simulink model "v1bate3"  (Simulink 8.8)
settings: Solver=ode3  StartTime=0.0  StopTime=inf  FixedStep=0.001  RelTol=1e-3  EnableMultiTasking=on
undefined symbols (not defined in the file): mdaadlink6208
libraries: simulink x19
(part 1 of 2)
settings Model: Creator=sayun  LastModifiedBy=lenovo  SimulationMode=external
settings SolverCC: EnableConcurrentExecution=on
settings OptimizationCC: BlockReduction=off  OptimizeBlockIOStorage=off  BufferReuse=off  GlobalBufferReuse=off  ExpressionFolding=off  ExpressionDepthLimit=2147483647  LocalBlockOutputs=off  LifeSpan=auto
settings DebuggingCC: SolverPrmCheckMsg=warning
settings HardwareCC: ProdIntDivRoundTo=Zero  ProdEndianess=LittleEndian  ProdLongLongMode=on  ProdHWDeviceType=Generic->32-bit x86 compatible
settings RTWCC: SystemTargetFile=slrt.tlc  TemplateMakefile=slrt_default_tmf  Description=Simulink Real-Time  RTWCompilerOptimization=on
settings SimulinkRealTimeCC: RL32LogBufSizeModifier=10000000

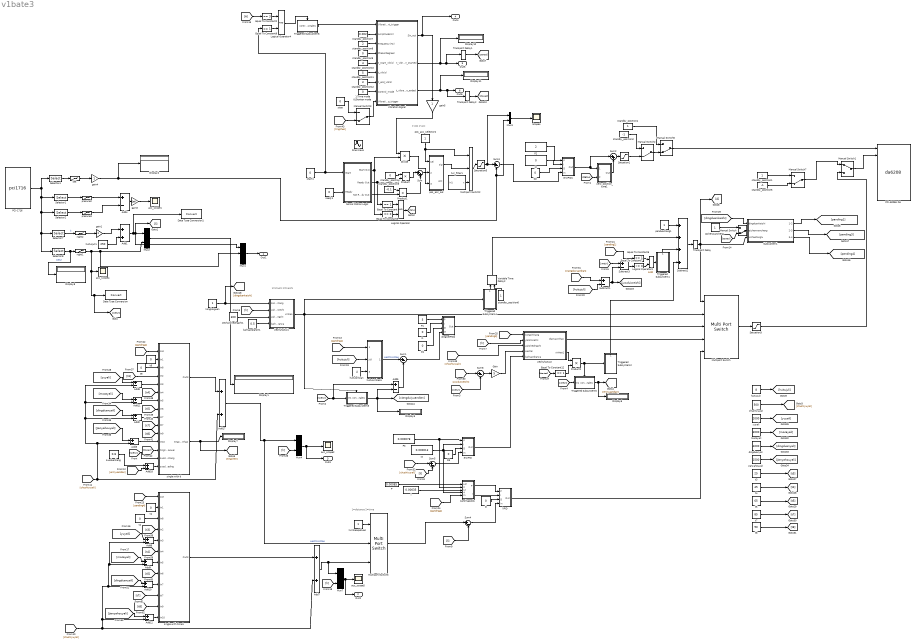
== system v1bate3 ==
  note: 1=chushi
      | 2=kaishi
  note: 1-pos
      | 2-acc
  note: 1=distance
      | 2=time
  1:Time mode 0:Shorten mode : Constant  Tag=kaognzhi  Description=kaognzhi  Value=0
  Add{1,7,17..18} (4 alike) : Sum
  Add{2..6,8..12} (10 alike) : Sum  Inputs=+-
  D{,1..3} (4 alike) : Constant  Value=0
  Data Type Conversion : DataTypeConversion
  Data Type Conversion1 : DataTypeConversion
  Display{1..2,5..8,10..11} (8 alike) : Display
  Divide : Product  Inputs=**
  Equal To Constant{,6,9,12} (4 alike) : simulink/Logic and Bit Operations/Compare To Constant  relop===  const=1  OutDataTypeStr=uint8  ZeroCross=off
  Equal To Constant2 : simulink/Logic and Bit Operations/Compare To Constant  relop===  const=3  OutDataTypeStr=uint8  ZeroCross=off
  Equal To Constant5 : simulink/Logic and Bit Operations/Compare To Constant  relop===  const=0  OutDataTypeStr=uint8  ZeroCross=off
  Equal To Constant7 : simulink/Logic and Bit Operations/Compare To Constant  relop=<=  const=0  OutDataTypeStr=uint8  ZeroCross=off
  Gain : Gain  Gain=5
  I : Constant  Value=0.00035
  I1 : Constant  Value=0
  I2 : Constant  Value=0
  I3 : Constant  Value=0.000013
  Logical Operator : Logic  AllPortsSameDT=off
  Logical Operator3 : Logic  AllPortsSameDT=off
  Logical Operator4 : Logic  AllPortsSameDT=off
  Manual Switch{,2..3,6..7} (5 alike) : ManualSwitch  CurrentSetting=0
  Manual Switch1 : ManualSwitch
  Multiport Switch : MultiPortSwitch  Inputs=4
  Multiport Switch2 : MultiPortSwitch  Inputs=2  SaturateOnIntegerOverflow=on
  Multiport Switch3 : MultiPortSwitch  Inputs=2
  Mux1 : Mux  Inputs=3
  Mux{2..4,7} (4 alike) : Mux  Inputs=2
  Nomal Motion Logic : Subsystem  AncestorBlock=control_logic_lib/Control Logic(Stateflow Chart)
  P : Constant  Value=0.00085
  P1 : Constant  Value=5
  P2 : Constant  Value=2
  P3 : Constant  Value=0.000078
  PCI-1716 : S-Function  FunctionName=pci1716  Parameters=[SampleTime SampleOffset], SLOT  SFunctionDeploymentMode=off  EnableBusSupport=off  mask(hitad3){Sample=0.001, SLOT=-1}
      mask prompts: Sample "Sample Time:"
      mask help:
      | PCi1716
      | A/D Card
      | Developed by ZhaoJinsong
      | 2012.06.02
      mask init:
      | SampleTime = 0.001; SampleOffset=0;
      mask Help: helpview([docroot '/toolbox/xpc/pt_io_block_reference.html#xpcioref'])
      mask Display:
      | disp('PCI1716  ');
      | 
      | port_label('output',1 , 'OUT');
  "PCI-6208A DA " : S-Function  InitFcn=mdaadlink6208( 1 );  FunctionName=da6208  Parameters=channel, range, sampletime, pcislot, reset, initval  SFunctionDeploymentMode=off  EnableBusSupport=off  mask(da6208){channel=[1:8], range=4 to 20 ma, reset=[0], initval=[0], sampletime=0.001, pcislot=-1}
      mask prompts: channel "Channel vector:"; reset "Reset vector:"; initval "Initial value vector:"; sampletime "Sample time:"; pcislot "PCI slot (-1: autosearch):"
      mask help:
      | PCI-6208A
      | Adlink
      | Analog Output
      mask init:
      | [maskdisplay, reset, initval]= mdaadlink6208(2, channel, reset, initval, pcislot);
      | set_param(gcb,'MaskDisplay',maskdisplay);
      mask Help: helpview(fullfile(docroot, 'mapfiles', 'xpc.map'), 'Adlink_6208A_DA')
      mask TypeOptions range: 0 to 20 ma | 5 to 25 ma | 4 to 20 ma
      mask Display: disp('PCI-6208A\nAdlink\nAnalog Output');port_label('input',1,'1');port_label('input',2,'2');port_label('input',3,'3');port_label('input',4,'4');port_label('input',5,'5');port_label('input',6,'6');port_label('input',7,'7');port_label('input',8,'8');
  Product : Product  SaturateOnIntegerOverflow=on  OutDataTypeStr=Inherit: Same as first input
  Product1 : Product  SaturateOnIntegerOverflow=on  OutDataTypeStr=Inherit: Same as first input
  Product2 : Product  RndMeth=Zero
  Satuation1 : Saturate  UpperLimit=10  LowerLimit=-10
  Satuation3 : Saturate  UpperLimit=10  LowerLimit=-10
  Saturation5 : Saturate  UpperLimit=10  LowerLimit=-10
  Scope4 : Scope
  Selector1 : Selector  IndexOptions=Index vector (dialog)  Indices=[3]  OutputSizes=1
  Selector2 : Selector  IndexOptions=Index vector (dialog)  Indices=[7]  OutputSizes=1
  Selector4 : Selector  IndexOptions=Index vector (dialog)  Indices=[1]  OutputSizes=1
  Selector7 : Selector  IndexOptions=Index vector (dialog)  Indices=[13]  OutputSizes=1
  Selector8 : Selector  IndexOptions=Index vector (dialog)  Indices=[15]  OutputSizes=1
  Sine Wave : Sin  Amplitude=0.001  Frequency=2*1*pi  SampleTime=0
  Subsystem1 : Subsystem
  Subtract1 : Sum  Inputs=+-
  Subtract2 : Sum  Inputs=++++
  Subtract3 : Sum  Inputs=+-
  Sum : Sum  Inputs=|++  SaturateOnIntegerOverflow=on
  Sum{1,4..5,8} (4 alike) : Sum  Inputs=|+-
  Sum2 : Sum  Inputs=|++  SaturateOnIntegerOverflow=on
  Sum3 : Sum  Inputs=|+-  SaturateOnIntegerOverflow=on
  Transport Delay : TransportDelay  DelayTime=0.0005
  Transport Delay1 : TransportDelay  DelayTime=0.0005
  Transport Delay2 : TransportDelay  DelayTime=0.0005
  Triggered Subsystem1 : Subsystem  TreatAsAtomicUnit=on
  Triggered Subsystem2 : Subsystem  TreatAsAtomicUnit=on
  Triggered Subsystem3 : Subsystem  TreatAsAtomicUnit=on
  Triggered Subsystem4 : Subsystem  TreatAsAtomicUnit=on
  Triggered Subsystem5 : Subsystem  TreatAsAtomicUnit=on
  Triggered Subsystem6 : Subsystem  TreatAsAtomicUnit=on
  Variable Time Delay2 : VariableTransportDelay  MaximumDelay=10
  Vibration Signal : Subsystem  TreatAsAtomicUnit=on
  acc_scope{1..2,4..5} (4 alike) : Scope
  canshuguodu : Subsystem
  chushiyuyali : Constant  Value=500
  dingduanyali : Constant  Value=4000
  dingweiPID2 : Subsystem
  erciPID : Subsystem
  erciPID1 : Subsystem
  gain1 : Gain  SaturateOnIntegerOverflow=on  OutDataTypeStr=Inherit: Same as input  ParamDataTypeStr=Inherit: Same as input
  gain3 : Gain  Gain=1e6  SaturateOnIntegerOverflow=on  OutDataTypeStr=Inherit: Same as input  ParamDataTypeStr=Inherit: Same as input
  gain4 : Gain  SaturateOnIntegerOverflow=on  OutDataTypeStr=Inherit: Same as input  ParamDataTypeStr=Inherit: Same as input
  gain5 : Gain  SaturateOnIntegerOverflow=on  OutDataTypeStr=Inherit: Same as input  ParamDataTypeStr=Inherit: Same as input
  huituijuli : Constant  Value=8
  huituijuli1 : Constant  Value=250
  huituishijian : Constant  Value=4
  huituixinhao1 : Subsystem
  jianyahouyali : Constant  Value=1500
  jiechuhuitui1 : Subsystem
  jiechuhuitui2 : Subsystem
  jiechulishedingzhi1 : Constant  Value=300
  kaihuanqianjin1 : Constant  Value=0.5
  left : Lookup  InputValues=[2.090 9.905]  Table=[-10 10]  SaturateOnIntegerOverflow=on
  liPID : Subsystem
  lixinhaoqiehuan : Constant
      settings: OpenFcn=|
      | if get_param(gcb,'value')=='1',
      | set_param(gcb,'value','2');
      | else
      | set_param(gcb,'value','1');end
  mocayali : Constant  Value=3000
  panduanliang1 : Constant
  pos_acc_sel : Subsystem
  pos_acc_selector2 : Constant
      settings: OpenFcn=|
      | if get_param(gcb,'value')=='1',
      | set_param(gcb,'value','2');
      | else
      | set_param(gcb,'value','1');end
  presure2 : Lookup  InputValues=[2 10]  Table=[0 25]  SaturateOnIntegerOverflow=on
  presure3 : Lookup  InputValues=[2 10]  Table=[0 25]  SaturateOnIntegerOverflow=on
  qizhenwancheng : Constant
      settings: OpenFcn=|
      | if get_param(gcb,'value')=='1',
      | set_param(gcb,'value','0');
      | else
      | set_param(gcb,'value','1');end
  ready1 : Constant  Value=0
      settings: OpenFcn=|
      | if get_param(gcb,'value')=='1',
      | set_param(gcb,'value','0');
      | else
      | set_param(gcb,'value','1');end
  right1 : Lookup  InputValues=[1.264 5.214]  Table=[0 20]  SaturateOnIntegerOverflow=on
  right2 : Lookup  InputValues=[2 10]  Table=[-29400 29400]  SaturateOnIntegerOverflow=on
  single with d : Subsystem
  single with time1 : Subsystem
  standby_position : Constant  Value=0
  standby_position1 : Constant
  standby_position10 : Constant  Value=4
  standby_position11 : Constant  Value=5
  standby_position12 : Constant  Value=3
  standby_position2 : Constant  Value=-1
  standby_position3 : Constant  Value=-0.1
  standby_position4 : Constant
  standby_position5 : Constant  Value=-1
  standby_position6 : Constant
  standby_position7 : Constant  Value=0.002
  standby_position8 : Constant  Value=2
  standby_position9 : Constant  Value=0
  start1 : Constant  Value=0
      settings: OpenFcn=|
      | if get_param(gcb,'value')=='1',
      | set_param(gcb,'value','0');
      | else
      | set_param(gcb,'value','1');end
  stop : Constant  Value=0
      settings: OpenFcn=|
      | if get_param(gcb,'value')=='1',
      | set_param(gcb,'value','0');
      | else
      | set_param(gcb,'value','1');end
  suoduanliang : Constant  Value=0.8
  t{1..2,6,9} (4 alike) : Constant  Value=0
  t3 : Constant  Value=25
  t4 : Constant  Value=45
  t5 : Constant  Value=65
  t7 : Constant  Value=85
  t8 : Constant  Value=90
  tvc_filter1 : Subsystem
      mask Display: disp('Reference\nModule')
  yuyali : Constant  Value=2000
  zero_position_tune1 : Subsystem
  zongkaiguan : Constant
      settings: OpenFcn=|
      | if get_param(gcb,'value')=='1',
      | set_param(gcb,'value','2');
      | else
      | set_param(gcb,'value','1');end
  Out1 : Outport
  Out2 : Outport  Port=2
  Out3 : Outport  Port=3
  Out4 : Outport  Port=4
  Out5 : Outport  Port=5
  Out6 : Outport  Port=6
  tag scope: status=global
  wires:
  kaihuanqianjin1/1 -> jiechuhuitui1/4(kaihuandianya)
  jiechulishedingzhi1/1 -> jiechuhuitui1/3(yalishedingzhi)
  jiechuhuitui1/1(xinhao) -> Triggered Subsystem4/Trigger, Triggered Subsystem3/Trigger, Multiport Switch/2
  huituishijian/1 -> huituixinhao1/3(shijian)
  [huitujuli] -> huituixinhao1/2(juli)
  panduanliang1/1 -> Subtract2/1
  Variable Time Delay2/1 -> Subtract2/2
  Equal To Constant7/1 -> Logical Operator3/2
  Equal To Constant6/1 -> Logical Operator3/1
  Subtract3/1 -> Equal To Constant7/1
  huituixinhao1/1(Out2) -> Sum1/1  "weizhixinhao"
  Sum1/1 -> dingweiPID2/4(In)
  zongkaiguan/1 -> [dingduankaishi], jiechuhuitui1/1(kongzhiliang)
  left/1 -> gain4/1
  PCI-1716/1 -> Selector4/1, Selector1/1, Selector2/1, Selector7/1, Selector8/1
  Selector4/1 -> left/1
  Selector1/1 -> presure2/1
  Selector2/1 -> presure3/1
  presure2/1 -> Add4/1
  presure3/1 -> Add4/2
  Add4/1 -> gain3/1
  gain3/1 -> acc_scope1/1
  Mux2/1 -> Display1/1
  Selector7/1 -> right2/1  "li"
  Selector8/1 -> right1/1, Display8/1  "weiyi"
  right2/1 -> gain1/1
  right1/1 -> Mux2/2, Mux1/2, acc_scope4/1, Data Type Conversion/1, [weiyi]
  gain1/1 -> Add1/1
  ready1/1 -> Nomal Motion Logic/2(Ready)
  start1/1 -> Nomal Motion Logic/1(Start), Equal To Constant9/1
  Nomal Motion Logic/2(Ready Out) -> Equal To Constant/1, Product/2
  standby_position/1 -> Product/1
  Product/1 -> Sum/1
  Sum/1 -> pos_acc_sel/3(ini_pos)
  Nomal Motion Logic/1(Start Out) -> Divide/2, Equal To Constant5/1
  Equal To Constant/1 -> Logical Operator/1
  Logical Operator/1 -> [status]
  pos_acc_selector2/1 -> pos_acc_sel/1(sel), Multiport Switch2/1
  Nomal Motion Logic/3(Not Ready Out) -> Product1/2
  standby_position3/1 -> Product1/1
  Product1/1 -> Sum/2
  Multiport Switch2/1 -> Saturation5/1
  [status] -> zero_position_tune1/2(status)
  pos_acc_sel/1(sig) -> Multiport Switch2/2
  zero_position_tune1/1(Out) -> Sum2/2
  Sum2/1 -> Satuation1/1
  Sum3/1 -> erciPID1/4(In)
  tvc_filter1/1(x) -> Multiport Switch2/3
  Satuation1/1 -> Manual Switch2/2
  standby_position2/1 -> Manual Switch2/1
  Saturation5/1 -> Sum3/1, Mux3/1
  Manual Switch2/1 -> Manual Switch6/2
  standby_position4/1 -> Manual Switch6/1
  Divide/1 -> pos_acc_sel/2(sig_in)
  erciPID1/1(Out) -> Sum2/1, zero_position_tune1/1(error_in)
  Mux3/1 -> Scope4/1
  Equal To Constant5/1 -> Logical Operator/2
  Manual Switch6/1 -> "PCI-6208A DA "/1
  gain4/1 -> Sum3/2, Mux3/2, Display2/1
  standby_position1/1 -> Manual Switch7/1
  standby_position5/1 -> Manual Switch7/2
  dingweiPID2/1(Out) -> Multiport Switch/3
  huituijuli1/1 -> Add1/2
  Add1/1 -> Data Type Conversion1/1, Mux2/1, [li], Mux1/1
  Mux1/1 -> Out1/1
  Transport Delay/1 -> [A], Subsystem1/3(xinhaotonglu), Multiport Switch/1
  Add5/1 -> Sum1/2
  chushiyuyali/1 -> [chushiyuyali]
  lixinhaoqiehuan/1 -> Multiport Switch3/1
  Logical Operator3/1 -> Triggered Subsystem1/Trigger
  Triggered Subsystem1/1(control-single1) -> Subtract2/3
  Product2/1 -> Triggered Subsystem2/Trigger, Triggered Subsystem5/Trigger
  single with time1/1(Out3) -> Add7/1
  Add7/1 -> Mux7/1, Multiport Switch3/3
  Triggered Subsystem2/1(control-single1) -> Subtract2/4
  canshuguodu/1(P) -> liPID/1(P)
  [yuyali] -> Add6/1
  Add6/1 -> single with time1/5(In3)
  Add9/1 -> single with time1/7(In5)
  Add10/1 -> single with time1/9(In7)
  P3/1 -> erciPID/1(P), canshuguodu/2(erciP)
  t1/1 -> single with time1/2(In1)
  t2/1 -> single with time1/3(In8)
  Add12/1 -> single with time1/12(In10)
  jiechuhuitui2/2(xinhao1) -> Product2/1
  I3/1 -> erciPID/2(I), canshuguodu/4(erciI)
  P/1 -> canshuguodu/1(LiP)
  I/1 -> canshuguodu/3(LiI)
  canshuguodu/2(I) -> liPID/2(I)
  Subtract1/1 -> Subtract3/2, [juwduiweizhi]
  Triggered Subsystem4/1(control-single1) -> Variable Time Delay2/1
  standby_position6/1 -> Variable Time Delay2/2
  t6/1 -> single with d/2(In1)
  single with d/1(Out3) -> Add17/1
  t9/1 -> single with d/3(In8)
  [stoped] -> single with d/13(tingzhendaowei)
  Add18/1 -> single with d/15(suoduanliangsheding)
  suoduanliang/1 -> Add18/1
  single with d/2(tingzhenxinhao) -> Display7/1, [tingzhen]
  Gain/1 -> jiechuhuitui2/4(wentai)
  Sum8/1 -> Gain/1
  standby_position7/1 -> Vibration Signal/2(Amplitude(m))
  standby_position8/1 -> Vibration Signal/3(Frequency(Hz))
  standby_position9/1 -> Vibration Signal/4(Phase(Degree))
  standby_position10/1 -> Vibration Signal/5(t_start_vib(s))
  Triggered Subsystem6/1(control-single1) -> Vibration Signal/1(Vibration_start_trigger)
  standby_position11/1 -> Vibration Signal/6(t_vib(s))
  standby_position12/1 -> Vibration Signal/7(t_end_vib(s))
  Vibration Signal/1(Sin_out) -> Out4/1, gain5/1
  Vibration Signal/2(t_vibration_started) -> Display10/1, Out5/1, Transport Delay1/1
  Vibration Signal/3(t_vibration_ended) -> Display11/1, Out6/1, Transport Delay2/1
  1:Time mode 0:Shorten mode/1 -> Vibration Signal/8(Control_mode)
  [weiyi] -> single with d/14(suoduanliang)
  [weiyi] -> Triggered Subsystem3/1(In1), Add5/1
  [weiyi] -> Sum8/2
  [weiyi] -> Triggered Subsystem5/1(In1)
  [weiyi] -> Subtract3/1
  [li] -> jiechuhuitui1/2(yalishicezhi)
  [li] -> jiechuhuitui2/2(yalishicezhi)
  [li] -> Sum5/2
  erciPID/1(Out) -> jiechuhuitui2/5(kaihuandianya)
  D3/1 -> erciPID/3(D)
  D/1 -> liPID/3(D)
  [chushiyuyali] -> Add7/2, Add12/2, Add10/2, Add9/2, Add6/2
  [chushiyuyali] -> Add17/2, Add3/2, Add2/2, Add11/2, Add8/2
  [erciyuandian] -> Add18/2
  gain5/1 -> Divide/1
  qizhenwancheng/1 -> Manual Switch/1
  [started] -> Manual Switch/2
  [A] -> Equal To Constant2/1
  Equal To Constant2/1 -> Logical Operator4/1
  Equal To Constant9/1 -> Logical Operator4/2
  Logical Operator4/1 -> Triggered Subsystem6/Trigger
  P2/1 -> erciPID1/1(P)
  I2/1 -> erciPID1/2(I)
  D2/1 -> erciPID1/3(D)
  huituijuli/1 -> [huitujuli]
  [huitujuli] -> Subtract1/2
  [panding4] -> single with d/1(con)
  [panding4] -> single with time1/1(con)
  [panding4] -> canshuguodu/5(In)
  [panding3] -> jiechuhuitui2/1(kongzhiliang)
  [started] -> Equal To Constant12/1
  Equal To Constant12/1 -> Product2/2
  [dingduankaishi] -> Subsystem1/1(dingduankaishi)
  Manual Switch/1 -> Subsystem1/2(qizhenwancheng)
  Subtract2/1 -> Transport Delay/1
  [juwduiweizhi] -> Sum8/1
  P1/1 -> dingweiPID2/1(P)
  I1/1 -> dingweiPID2/2(I)
  D1/1 -> dingweiPID2/3(D)
  [xiangduiyuandian] -> Subtract1/1
  Triggered Subsystem5/1(control-single1) -> [erciyuandian], Display6/1
  Triggered Subsystem3/1(control-single1) -> Add5/2, [xiangduiyuandian], Display5/1
  [chushiyuyali] -> Sum5/1
  [chushiyuyali] -> jiechuhuitui2/3(yalishedingzhi)
  Sum5/1 -> erciPID/4(In)
  ? -> ?
  [t3] -> single with time1/4(In2)
  [mocayali] -> Add9/1
  [dingduanyali] -> Add10/1
  [jianyahouyali] -> Add12/1
  [li] -> Sum4/2
  Sum4/1 -> liPID/4(In)
  Multiport Switch3/1 -> Sum4/1
  Mux7/1 -> acc_scope5/1, Out2/1
  [li] -> Mux7/2
  Mux4/1 -> acc_scope2/1, Out3/1
  [li] -> Mux4/2
  [t4] -> single with time1/6(In4)
  [t5] -> single with time1/8(In6)
  [t7] -> single with time1/10(tt7)
  [t8] -> single with time1/11(In9)
  [yuyali] -> Add8/1
  [mocayali] -> Add11/1
  [dingduanyali] -> Add2/1
  [jianyahouyali] -> Add3/1
  Add3/1 -> single with d/12(In10)
  [t3] -> single with d/4(In2)
  Add8/1 -> single with d/5(In3)
  [t4] -> single with d/6(In4)
  Add11/1 -> single with d/7(In5)
  [t5] -> single with d/8(In6)
  Add2/1 -> single with d/9(In7)
  [t7] -> single with d/10(tt7)
  [t8] -> single with d/11(In9)
  Add17/1 -> Mux4/1, Multiport Switch3/2  "weizhixinhao"
  yuyali/1 -> [yuyali]
  mocayali/1 -> [mocayali]
  dingduanyali/1 -> [dingduanyali]
  jianyahouyali/1 -> [jianyahouyali]
  t3/1 -> [t3]
  t4/1 -> [t4]
  t5/1 -> [t5]
  t7/1 -> [t7]
  t8/1 -> [t8]
  Manual Switch7/1 -> Manual Switch1/1
  [panding1] -> Equal To Constant6/1
  Subsystem1/1(1-2) -> [panding1]
  Subsystem1/2(2-3) -> [panding3]
  Subsystem1/3(3-4) -> [panding4]
  Multiport Switch/1 -> Satuation3/1
  jiechuhuitui2/1(dianyaxinhao) -> Multiport Switch/4
  [panding1] -> huituixinhao1/1(con1)
  liPID/1(Out) -> Multiport Switch/5
  Manual Switch1/1 -> "PCI-6208A DA "/2
  Satuation3/1 -> Manual Switch1/2
  Manual Switch3/1 -> Vibration Signal/9(Vibration_stop_trigger)
  stop/1 -> Manual Switch3/1
  [tingzhen] -> Manual Switch3/2
  Transport Delay2/1 -> [stoped]
  Transport Delay1/1 -> [started]

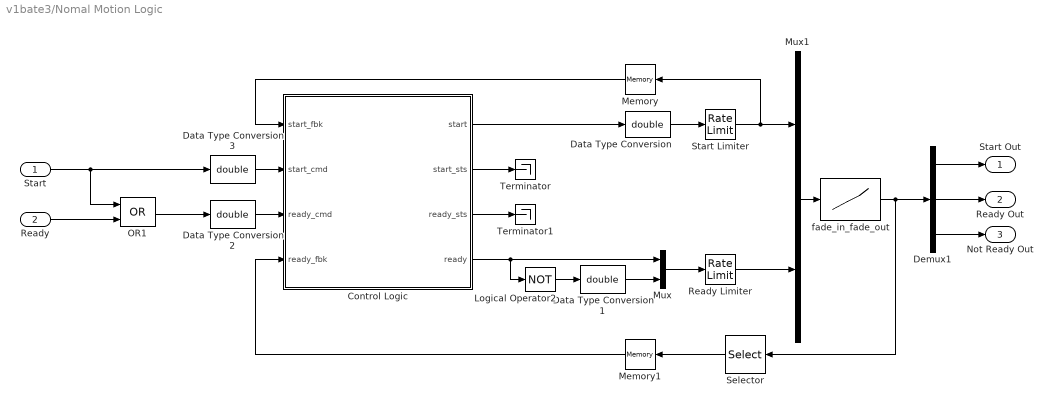
== system v1bate3/Nomal Motion Logic ==
  Start : Inport
  Ready : Inport  Port=2
  Control Logic : Stateflow chart  TreatAsAtomicUnit=on
  Data Type Conversion{,1..3} (4 alike) : DataTypeConversion  OutDataTypeStr=double  SaturateOnIntegerOverflow=on  RndMeth=Zero
  Demux1 : Demux  Outputs=3
  Logical Operator2 : Logic  Operator=NOT  Inputs=3  AllPortsSameDT=off
  Memory : Memory
  Memory1 : Memory
  Mux : Mux  Inputs=2
  Mux1 : Mux  Inputs=2
  OR1 : Logic  Operator=OR  AllPortsSameDT=off
  Ready Limiter : RateLimiter  RisingSlewLimit=1/5  FallingSlewLimit=-1/5
  Selector : Selector  InputPortWidth=3  IndexOptions=Index vector (dialog)  Indices=[2]  OutputSizes=1
  Start Limiter : RateLimiter  RisingSlewLimit=1/3  FallingSlewLimit=-1/3
  Terminator : Terminator
  Terminator1 : Terminator
  fade_in_fade_out : Lookup  InputValues=[0:0.001:1]  Table=(sin(([0:0.001:1]*2-1)*pi/2)+1)/2  SaturateOnIntegerOverflow=on
  Start Out : Outport
  Ready Out : Outport  Port=2
  Not Ready Out : Outport  Port=3
  wires:
  Ready/1 -> OR1/2
  Start/1 -> OR1/1, Data Type Conversion3/1
  Control Logic/3(ready_sts) -> Terminator1/1
  Control Logic/2(start_sts) -> Terminator/1
  OR1/1 -> Data Type Conversion2/1
  Data Type Conversion3/1 -> Control Logic/2(start_cmd)
  Demux1/3 -> Not Ready Out/1
  Demux1/1 -> Start Out/1
  Demux1/2 -> Ready Out/1
  Data Type Conversion/1 -> Start Limiter/1
  Start Limiter/1 -> Mux1/1, Memory/1
  Control Logic/1(start) -> Data Type Conversion/1
  Control Logic/4(ready) -> Logical Operator2/1, Mux/1
  Logical Operator2/1 -> Data Type Conversion1/1
  Mux/1 -> Ready Limiter/1
  Ready Limiter/1 -> Mux1/2
  Mux1/1 -> fade_in_fade_out/1
  fade_in_fade_out/1 -> Selector/1, Demux1/1
  Memory/1 -> Control Logic/1(start_fbk)
  Memory1/1 -> Control Logic/4(ready_fbk)
  Data Type Conversion1/1 -> Mux/2
  Data Type Conversion2/1 -> Control Logic/3(ready_cmd)
  Selector/1 -> Memory1/1

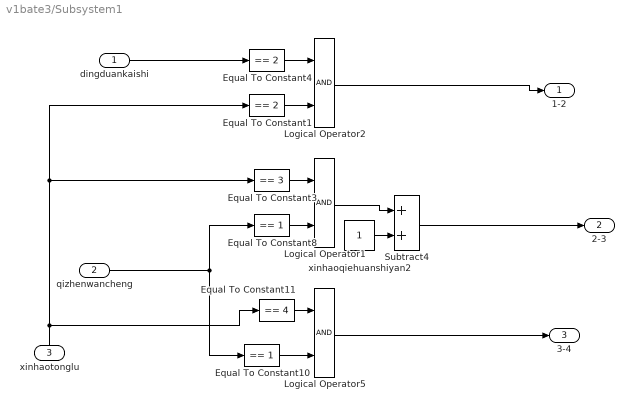
== system v1bate3/Subsystem1 ==
  dingduankaishi : Inport
  qizhenwancheng : Inport  Port=2
  xinhaotonglu : Inport  Port=3
  Equal To Constant1 : simulink/Logic and Bit Operations/Compare To Constant  relop===  const=2  OutDataTypeStr=uint8  ZeroCross=off
  Equal To Constant10 : simulink/Logic and Bit Operations/Compare To Constant  relop===  const=1  OutDataTypeStr=uint8  ZeroCross=off
  Equal To Constant11 : simulink/Logic and Bit Operations/Compare To Constant  relop===  const=4  OutDataTypeStr=uint8  ZeroCross=off
  Equal To Constant3 : simulink/Logic and Bit Operations/Compare To Constant  relop===  const=3  OutDataTypeStr=uint8  ZeroCross=off
  Equal To Constant4 : simulink/Logic and Bit Operations/Compare To Constant  relop===  const=2  OutDataTypeStr=uint8  ZeroCross=off
  Equal To Constant8 : simulink/Logic and Bit Operations/Compare To Constant  relop===  const=1  OutDataTypeStr=uint8  ZeroCross=off
  Logical Operator1 : Logic  AllPortsSameDT=off
  Logical Operator2 : Logic  AllPortsSameDT=off
  Logical Operator5 : Logic  AllPortsSameDT=off
  Subtract4 : Sum
  xinhaoqiehuanshiyan2 : Constant
  1-2 : Outport
  2-3 : Outport  Port=2
  3-4 : Outport  Port=3
  wires:
  Equal To Constant4/1 -> Logical Operator2/1
  Equal To Constant1/1 -> Logical Operator2/2
  Equal To Constant3/1 -> Logical Operator1/1
  Equal To Constant8/1 -> Logical Operator1/2
  xinhaoqiehuanshiyan2/1 -> Subtract4/2
  Logical Operator1/1 -> Subtract4/1
  Equal To Constant11/1 -> Logical Operator5/1
  Equal To Constant10/1 -> Logical Operator5/2
  qizhenwancheng/1 -> Equal To Constant10/1, Equal To Constant8/1
  xinhaotonglu/1 -> Equal To Constant11/1, Equal To Constant3/1, Equal To Constant1/1
  dingduankaishi/1 -> Equal To Constant4/1
  Logical Operator2/1 -> 1-2/1
  Subtract4/1 -> 2-3/1
  Logical Operator5/1 -> 3-4/1

== system v1bate3/Triggered Subsystem1 ==
  Trigger : TriggerPort  VariantControl=Variant
  Constant : Constant
  control-single1 : Outport
  wires:
  Constant/1 -> control-single1/1

== system v1bate3/Triggered Subsystem2 ==
  Trigger : TriggerPort  VariantControl=Variant
  Constant : Constant
  control-single1 : Outport
  wires:
  Constant/1 -> control-single1/1

== system v1bate3/Triggered Subsystem3 ==
  In1 : Inport
  Trigger : TriggerPort  TriggerType=falling  VariantControl=Variant
  control-single1 : Outport
  wires:
  In1/1 -> control-single1/1

== system v1bate3/Triggered Subsystem4 ==
  Trigger : TriggerPort  TriggerType=falling  VariantControl=Variant
  Constant : Constant
  control-single1 : Outport
  wires:
  Constant/1 -> control-single1/1

== system v1bate3/Triggered Subsystem5 ==
  In1 : Inport
  Trigger : TriggerPort  VariantControl=Variant
  control-single1 : Outport
  wires:
  In1/1 -> control-single1/1

== system v1bate3/Triggered Subsystem6 ==
  Trigger : TriggerPort  VariantControl=Variant
  Constant : Constant
  control-single1 : Outport
  wires:
  Constant/1 -> control-single1/1

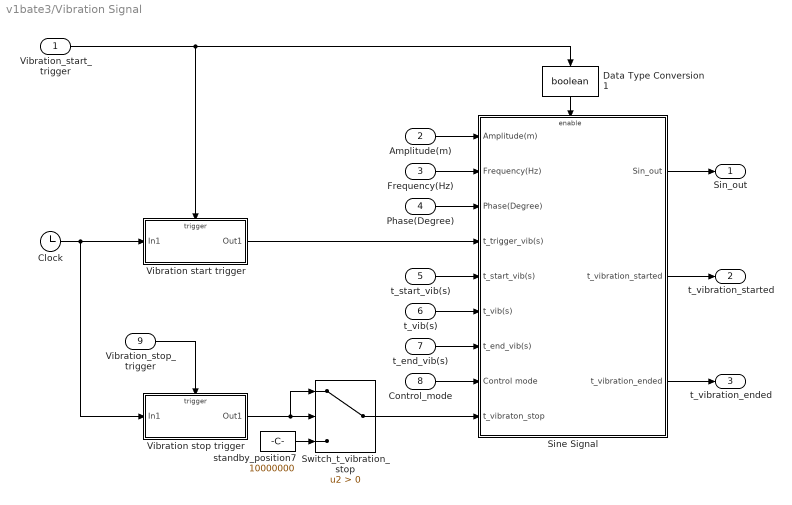
== system v1bate3/Vibration Signal ==
  Vibration_start_trigger : Inport
  Amplitude(m) : Inport  Port=2
  Frequency(Hz) : Inport  Port=3
  Phase(Degree) : Inport  Port=4
  t_start_vib(s) : Inport  Port=5
  t_vib(s) : Inport  Port=6
  t_end_vib(s) : Inport  Port=7
  Control_mode : Inport  Port=8
  Vibration_stop_trigger : Inport  Port=9
  Clock : Clock
  Data Type Conversion1 : DataTypeConversion  OutDataTypeStr=boolean  SaturateOnIntegerOverflow=on  RndMeth=Zero
  Sine Signal : Subsystem
  Switch_t_vibration_stop : Switch  Criteria=u2 > Threshold
  Vibration start trigger : Subsystem  TreatAsAtomicUnit=on
  Vibration stop trigger : Subsystem  TreatAsAtomicUnit=on
  standby_position7 : Constant  Value=10000000
  Sin_out : Outport
  t_vibration_started : Outport  Port=2
  t_vibration_ended : Outport  Port=3
  wires:
  Data Type Conversion1/1 -> Sine Signal/Enable
  Phase(Degree)/1 -> Sine Signal/3(Phase(Degree))
  Vibration_start_trigger/1 -> Data Type Conversion1/1, Vibration start trigger/Trigger
  Frequency(Hz)/1 -> Sine Signal/2(Frequency(Hz))
  Vibration start trigger/1(Out1) -> Sine Signal/4(t_trigger_vib(s))
  Clock/1 -> Vibration start trigger/1(In1), Vibration stop trigger/1(In1)
  Amplitude(m)/1 -> Sine Signal/1(Amplitude(m))
  t_start_vib(s)/1 -> Sine Signal/5(t_start_vib(s))
  t_vib(s)/1 -> Sine Signal/6(t_vib(s))
  t_end_vib(s)/1 -> Sine Signal/7(t_end_vib(s))
  Sine Signal/1(Sin_out) -> Sin_out/1
  Sine Signal/2(t_vibration_started) -> t_vibration_started/1
  Sine Signal/3(t_vibration_ended) -> t_vibration_ended/1
  Control_mode/1 -> Sine Signal/8(Control mode)
  Vibration_stop_trigger/1 -> Vibration stop trigger/Trigger
  standby_position7/1 -> Switch_t_vibration_stop/3
  Vibration stop trigger/1(Out1) -> Switch_t_vibration_stop/2, Switch_t_vibration_stop/1
  Switch_t_vibration_stop/1 -> Sine Signal/9(t_vibraton_stop)

== system v1bate3/canshuguodu ==
  LiP : Inport
  erciP : Inport  Port=2
  LiI : Inport  Port=3
  erciI : Inport  Port=4
  In : Inport  Port=5
  Nomal Motion Logic1 : Subsystem  AncestorBlock=control_logic_lib/Control Logic(Stateflow Chart)
  Nomal Motion Logic2 : Subsystem  AncestorBlock=control_logic_lib/Control Logic(Stateflow Chart)
  Product{12..15} (4 alike) : Product  SaturateOnIntegerOverflow=on  OutDataTypeStr=Inherit: Same as first input
  Sum6 : Sum  Inputs=|++  SaturateOnIntegerOverflow=on
  Sum7 : Sum  Inputs=|++  SaturateOnIntegerOverflow=on
  start4 : Constant  Value=0
      settings: OpenFcn=|
      | if get_param(gcb,'value')=='1',
      | set_param(gcb,'value','0');
      | else
      | set_param(gcb,'value','1');end
  start5 : Constant  Value=0
      settings: OpenFcn=|
      | if get_param(gcb,'value')=='1',
      | set_param(gcb,'value','0');
      | else
      | set_param(gcb,'value','1');end
  P : Outport
  I : Outport  Port=2
  wires:
  start4/1 -> Nomal Motion Logic1/1(Start)
  Nomal Motion Logic1/2(Ready Out) -> Product12/2
  Product12/1 -> Sum6/1
  Nomal Motion Logic1/3(Not Ready Out) -> Product13/2
  Product13/1 -> Sum6/2
  start5/1 -> Nomal Motion Logic2/1(Start)
  Nomal Motion Logic2/2(Ready Out) -> Product14/2
  Product14/1 -> Sum7/1
  Nomal Motion Logic2/3(Not Ready Out) -> Product15/2
  Product15/1 -> Sum7/2
  erciP/1 -> Product13/1
  In/1 -> Nomal Motion Logic2/2(Ready), Nomal Motion Logic1/2(Ready)
  erciI/1 -> Product15/1
  Nomal Motion Logic1/1(Start Out) -> ?
  LiP/1 -> Product12/1
  Sum6/1 -> P/1
  Nomal Motion Logic2/1(Start Out) -> ?
  LiI/1 -> Product14/1
  Sum7/1 -> I/1

== system v1bate3/dingweiPID2 ==
  P : Inport
  I : Inport  Port=2
  D : Inport  Port=3
  In : Inport  Port=4
  Add19 : Sum  Inputs=+++
  Derivative4 : Derivative
  Integrator5 : Integrator
  Product16 : Product  RndMeth=Zero
  Product17 : Product  RndMeth=Zero
  Product18 : Product  RndMeth=Zero
  Out : Outport
  wires:
  D/1 -> Product17/1
  Add19/1 -> Out/1
  I/1 -> Product16/1
  In/1 -> Product17/2, Product16/2, Product18/2
  P/1 -> Product18/1
  Product17/1 -> Derivative4/1
  Product16/1 -> Integrator5/1
  Product18/1 -> Add19/1
  Integrator5/1 -> Add19/2
  Derivative4/1 -> Add19/3

== system v1bate3/erciPID ==
  P : Inport
  I : Inport  Port=2
  D : Inport  Port=3
  In : Inport  Port=4
  Add19 : Sum  Inputs=+++
  Derivative4 : Derivative
  Integrator5 : Integrator
  Product16 : Product  RndMeth=Zero
  Product17 : Product  RndMeth=Zero
  Product18 : Product  RndMeth=Zero
  Out : Outport
  wires:
  Derivative4/1 -> Add19/3
  Integrator5/1 -> Add19/2
  Product18/1 -> Add19/1
  Product16/1 -> Integrator5/1
  Product17/1 -> Derivative4/1
  P/1 -> Product18/1
  In/1 -> Product18/2, Product16/2, Product17/2
  I/1 -> Product16/1
  Add19/1 -> Out/1
  D/1 -> Product17/1

== system v1bate3/erciPID1 ==
  P : Inport
  I : Inport  Port=2
  D : Inport  Port=3
  In : Inport  Port=4
  Add19 : Sum  Inputs=+++
  Derivative4 : Derivative
  Integrator5 : Integrator
  Product16 : Product  RndMeth=Zero
  Product17 : Product  RndMeth=Zero
  Product18 : Product  RndMeth=Zero
  Out : Outport
  wires:
  D/1 -> Product17/1
  Add19/1 -> Out/1
  I/1 -> Product16/1
  In/1 -> Product17/2, Product16/2, Product18/2
  P/1 -> Product18/1
  Product17/1 -> Derivative4/1
  Product16/1 -> Integrator5/1
  Product18/1 -> Add19/1
  Integrator5/1 -> Add19/2
  Derivative4/1 -> Add19/3

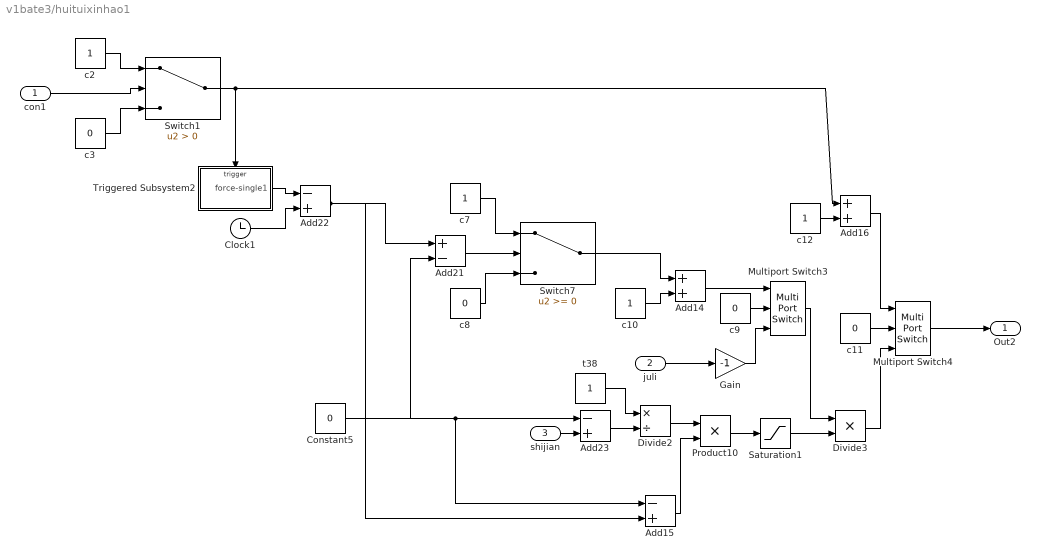
== system v1bate3/huituixinhao1 ==
  con1 : Inport
  juli : Inport  Port=2
  shijian : Inport  Port=3
  Add14 : Sum
  Add15 : Sum  Inputs=-+
  Add16 : Sum
  Add21 : Sum  Inputs=+-
  Add22 : Sum  Inputs=-+
  Add23 : Sum  Inputs=-+
  Clock1 : Clock
  Constant5 : Constant  Value=0
  Divide2 : Product  Inputs=*/
  Divide3 : Product  Inputs=**
  Gain : Gain  Gain=-1
  Multiport Switch3 : MultiPortSwitch  Inputs=2
  Multiport Switch4 : MultiPortSwitch  Inputs=2
  Product10 : Product  RndMeth=Zero
  Saturation1 : Saturate  UpperLimit=1  LowerLimit=-1
  Switch1 : Switch  Criteria=u2 > Threshold
  Switch7 : Switch
  Triggered Subsystem2 : Subsystem  TreatAsAtomicUnit=on
  c{2,7,10,12} (4 alike) : Constant
  c{3,8..9,11} (4 alike) : Constant  Value=0
  t38 : Constant
  Out2 : Outport
  wires:
  c12/1 -> Add16/2
  Multiport Switch4/1 -> Out2/1
  Add16/1 -> Multiport Switch4/1
  c11/1 -> Multiport Switch4/2
  shijian/1 -> Add23/2
  juli/1 -> Gain/1
  con1/1 -> Switch1/2
  Gain/1 -> Multiport Switch3/3
  Switch1/1 -> Add16/1, Triggered Subsystem2/Trigger
  c3/1 -> Switch1/3
  c2/1 -> Switch1/1
  Add22/1 -> Add15/2, Add21/1
  c10/1 -> Add14/2
  Switch7/1 -> Add14/1
  Add14/1 -> Multiport Switch3/1
  c9/1 -> Multiport Switch3/2
  Add21/1 -> Switch7/2
  c8/1 -> Switch7/3
  c7/1 -> Switch7/1
  Multiport Switch3/1 -> Divide3/1
  Constant5/1 -> Add21/2, Add15/1, Add23/1
  Add15/1 -> Product10/2
  Divide2/1 -> Product10/1
  Add23/1 -> Divide2/2
  Saturation1/1 -> Divide3/2
  Product10/1 -> Saturation1/1
  t38/1 -> Divide2/1
  Clock1/1 -> Add22/2
  Triggered Subsystem2/1(force-single1) -> Add22/1
  Divide3/1 -> Multiport Switch4/3

== system v1bate3/jiechuhuitui1 ==
  kongzhiliang : Inport
  yalishicezhi : Inport  Port=2
  yalishedingzhi : Inport  Port=3
  kaihuandianya : Inport  Port=4
  Add : Sum  Inputs=+-
  Add1 : Sum  Inputs=+-
  Multiport Switch : MultiPortSwitch
  Switch1 : Switch
  c2 : Constant  Value=-1
  c3 : Constant  Value=0
  chushi : Constant  Value=-1
  tingzhi : Constant  Value=0
  xinhao : Outport
  wires:
  chushi/1 -> Multiport Switch/2
  c2/1 -> Switch1/1
  c3/1 -> Switch1/3
  Add/1 -> Switch1/2
  tingzhi/1 -> Multiport Switch/4
  Switch1/1 -> Add1/2
  Add1/1 -> Multiport Switch/1
  kongzhiliang/1 -> Add1/1
  yalishicezhi/1 -> Add/1
  yalishedingzhi/1 -> Add/2
  kaihuandianya/1 -> Multiport Switch/3
  Multiport Switch/1 -> xinhao/1  "dianya"

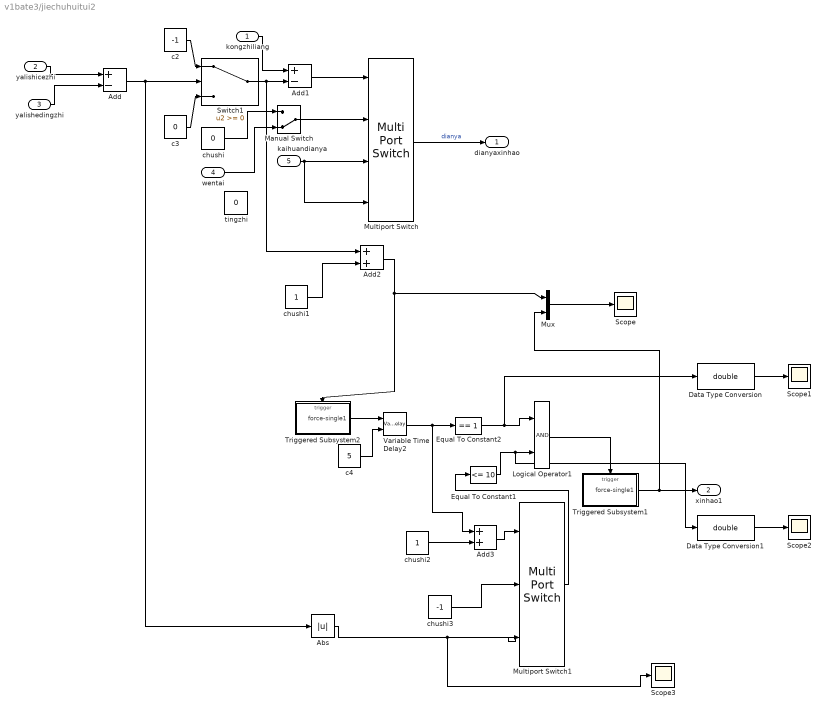
== system v1bate3/jiechuhuitui2 ==
  kongzhiliang : Inport
  yalishicezhi : Inport  Port=2
  yalishedingzhi : Inport  Port=3
  wentai : Inport  Port=4
  kaihuandianya : Inport  Port=5
  Abs : Abs
  Add : Sum  Inputs=+-
  Add1 : Sum  Inputs=+-
  Add2 : Sum
  Add3 : Sum
  Data Type Conversion : DataTypeConversion  OutDataTypeStr=double
  Data Type Conversion1 : DataTypeConversion  OutDataTypeStr=double
  Equal To Constant1 : simulink/Logic and Bit Operations/Compare To Constant  relop=<=  const=10  OutDataTypeStr=uint8  ZeroCross=off
  Equal To Constant2 : simulink/Logic and Bit Operations/Compare To Constant  relop===  const=1  OutDataTypeStr=uint8  ZeroCross=off
  Logical Operator1 : Logic  AllPortsSameDT=off
  Manual Switch : ManualSwitch  CurrentSetting=0
  Multiport Switch : MultiPortSwitch
  Multiport Switch1 : MultiPortSwitch  Inputs=2
  Mux : Mux  Inputs=2
  Scope{,1..3} (4 alike) : Scope
  Switch1 : Switch
  Triggered Subsystem1 : Subsystem  TreatAsAtomicUnit=on
  Triggered Subsystem2 : Subsystem  TreatAsAtomicUnit=on
  Variable Time Delay2 : VariableTransportDelay  MaximumDelay=10
  c2 : Constant  Value=-1
  c3 : Constant  Value=0
  c4 : Constant  Value=5
  chushi : Constant  Value=0
  chushi1 : Constant
  chushi2 : Constant
  chushi3 : Constant  Value=-1
  tingzhi : Constant  Value=0
  dianyaxinhao : Outport
  xinhao1 : Outport  Port=2
  wires:
  Multiport Switch/1 -> dianyaxinhao/1  "dianya"
  yalishedingzhi/1 -> Add/2
  yalishicezhi/1 -> Add/1
  kongzhiliang/1 -> Add1/1
  Add1/1 -> Multiport Switch/1
  Switch1/1 -> Add1/2, Add2/1
  Add/1 -> Switch1/2, Abs/1
  c3/1 -> Switch1/3
  c2/1 -> Switch1/1
  chushi/1 -> Manual Switch/1
  wentai/1 -> Manual Switch/2
  Manual Switch/1 -> Multiport Switch/2
  kaihuandianya/1 -> Multiport Switch/3, Multiport Switch/4
  chushi1/1 -> Add2/2
  Add2/1 -> Triggered Subsystem2/Trigger, Mux/1
  Triggered Subsystem2/1(force-single1) -> Variable Time Delay2/1
  Equal To Constant1/1 -> Logical Operator1/2, Data Type Conversion1/1
  Triggered Subsystem1/1(force-single1) -> xinhao1/1, Mux/2
  Logical Operator1/1 -> Triggered Subsystem1/Trigger
  Variable Time Delay2/1 -> Add3/1, Equal To Constant2/1
  c4/1 -> Variable Time Delay2/2
  Mux/1 -> Scope/1
  chushi2/1 -> Add3/2
  Abs/1 -> Multiport Switch1/3, Scope3/1
  Add3/1 -> Multiport Switch1/1
  chushi3/1 -> Multiport Switch1/2
  Multiport Switch1/1 -> Equal To Constant1/1
  Equal To Constant2/1 -> Logical Operator1/1, Data Type Conversion/1
  Data Type Conversion/1 -> Scope1/1
  Data Type Conversion1/1 -> Scope2/1

== system v1bate3/liPID ==
  P : Inport
  I : Inport  Port=2
  D : Inport  Port=3
  In : Inport  Port=4
  Add19 : Sum  Inputs=+++
  Derivative4 : Derivative
  Integrator5 : Integrator
  Product16 : Product  RndMeth=Zero
  Product17 : Product  RndMeth=Zero
  Product18 : Product  RndMeth=Zero
  Out : Outport
  wires:
  D/1 -> Product17/1
  Add19/1 -> Out/1
  I/1 -> Product16/1
  In/1 -> Product17/2, Product16/2, Product18/2
  P/1 -> Product18/1
  Product17/1 -> Derivative4/1
  Product16/1 -> Integrator5/1
  Product18/1 -> Add19/1
  Integrator5/1 -> Add19/2
  Derivative4/1 -> Add19/3

== system v1bate3/pos_acc_sel ==
  note: g
  note: V
  sel : Inport
  sig_in : Inport  Port=2
  ini_pos : Inport  Port=3
  Discrete inverse fit : DiscreteTransferFcn  Numerator=[1 -5.513868347662695 12.88491366007906 -16.323990002559352 11.821537968329908 -4.639485908156727 0.77101716333547]  Denominator=[0.013392688630559 -0.043519228995354 0.057088791124972 -0.038794303856191 0.015270049598488 -0.003637012524308 0.000292524753671]  SampleTime=0.001
  Multiport Switch : MultiPortSwitch  Inputs=2  SaturateOnIntegerOverflow=on
  Multiport Switch1 : MultiPortSwitch  Inputs=2  SaturateOnIntegerOverflow=on
  Product : Product  SaturateOnIntegerOverflow=on  OutDataTypeStr=Inherit: Same as first input
  Product1 : Product  SaturateOnIntegerOverflow=on  OutDataTypeStr=Inherit: Same as first input
  Sum1 : Sum  Inputs=|++  SaturateOnIntegerOverflow=on
  internal_sig_acc_gain : Constant
  internal_sig_pos_gain : Constant  Value=20/0.2
  "sel " : Constant
  sig : Outport
  acc : Outport  Port=2
  wires:
  internal_sig_acc_gain/1 -> Product1/1
  Product1/1 -> Discrete inverse fit/1, Multiport Switch1/2, acc/1
  internal_sig_pos_gain/1 -> Product/1
  Product/1 -> Multiport Switch/2
  Sum1/1 -> Product/2
  ini_pos/1 -> Sum1/2
  Multiport Switch/1 -> sig/1
  sel/1 -> Multiport Switch/1
  sig_in/1 -> Product1/2, Sum1/1
  Discrete inverse fit/1 -> Multiport Switch1/3
  "sel "/1 -> Multiport Switch1/1
  Multiport Switch1/1 -> Multiport Switch/3

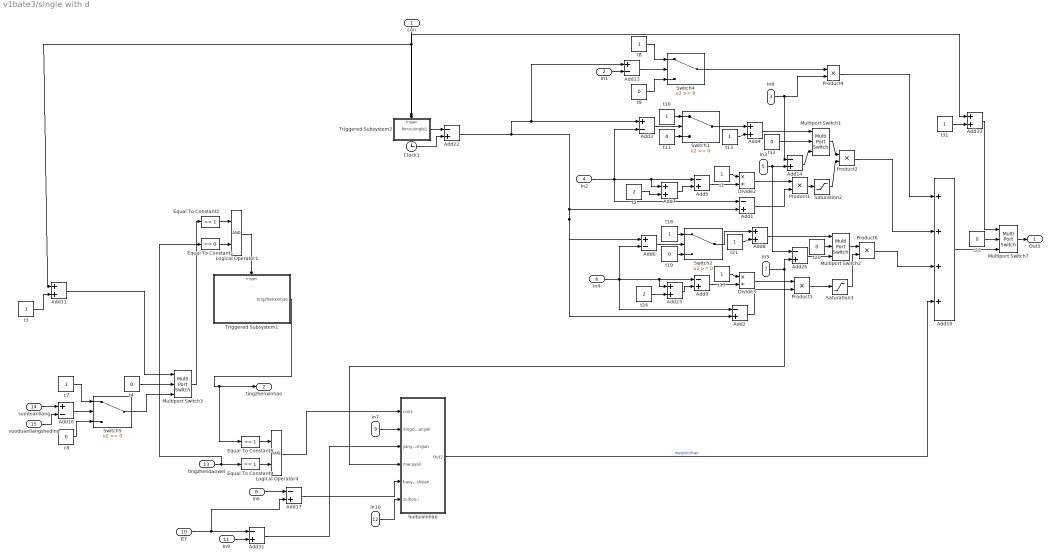
== system v1bate3/single with d ==
  con : Inport
  In1 : Inport  Port=2
  In8 : Inport  Port=3
  In2 : Inport  Port=4
  In3 : Inport  Port=5
  In4 : Inport  Port=6
  In5 : Inport  Port=7
  In6 : Inport  Port=8
  In7 : Inport  Port=9
  tt7 : Inport  Port=10
  In9 : Inport  Port=11
  In10 : Inport  Port=12
  tingzhendaowei : Inport  Port=13
  suoduanliang : Inport  Port=14
  suoduanliangsheding : Inport  Port=15
  Add{1..2,5,9,14,17,22,26,31} (9 alike) : Sum  Inputs=-+
  Add10 : Sum  Inputs=++++
  Add{4,7..8,11,23,33} (6 alike) : Sum
  Add{3,6,13,16} (4 alike) : Sum  Inputs=+-
  Clock1 : Clock
  Divide2 : Product  Inputs=*/
  Divide3 : Product  Inputs=*/
  Equal To Constant1 : simulink/Logic and Bit Operations/Compare To Constant  relop===  const=0  OutDataTypeStr=uint8  ZeroCross=off
  Equal To Constant2 : simulink/Logic and Bit Operations/Compare To Constant  relop===  const=1  OutDataTypeStr=uint8  ZeroCross=off
  Equal To Constant8 : simulink/Logic and Bit Operations/Compare To Constant  relop===  const=1  OutDataTypeStr=uint8  ZeroCross=off
  Equal To Constant9 : simulink/Logic and Bit Operations/Compare To Constant  relop===  const=1  OutDataTypeStr=uint8  ZeroCross=off
  Logical Operator1 : Logic  AllPortsSameDT=off
  Logical Operator4 : Logic  AllPortsSameDT=off
  Multiport Switch{1..3,7} (4 alike) : MultiPortSwitch  Inputs=2
  Product{1..3,6} (4 alike) : Product  RndMeth=Zero
  Product4 : Product  SaturateOnIntegerOverflow=on  OutDataTypeStr=Inherit: Same as first input
  Saturation2 : Saturate  UpperLimit=1  LowerLimit=-1
  Saturation3 : Saturate  UpperLimit=1  LowerLimit=-1
  Switch{1..2,4..5} (4 alike) : Switch
  Triggered Subsystem1 : Subsystem  TreatAsAtomicUnit=on
  Triggered Subsystem2 : Subsystem  TreatAsAtomicUnit=on
  c7 : Constant
  c8 : Constant  Value=0
  huituixinhao : Subsystem
  t{1,3,8,10,13,17..18,21,31} (9 alike) : Constant
  t{4,9,11..12,19..20,22} (7 alike) : Constant  Value=0
  t2 : Constant  Value=2
  t24 : Constant  Value=2
  Out3 : Outport
  tingzhenxinhao : Outport  Port=2
  wires:
  Add14/1 -> Multiport Switch1/3
  In8/1 -> Add14/1, Product4/2
  In1/1 -> Add13/2
  Product4/1 -> Add10/1
  Switch4/1 -> Product4/1
  Add13/1 -> Switch4/2
  t9/1 -> Switch4/3
  t8/1 -> Switch4/1
  t2/1 -> Add7/2
  Add7/1 -> Add5/2
  Add22/1 -> Add13/1, Add3/1, Add1/2, Add6/1, Add2/2
  Add10/1 -> Multiport Switch7/3
  t22/1 -> Multiport Switch7/2
  Add33/1 -> Multiport Switch7/1
  Multiport Switch7/1 -> Out3/1
  t31/1 -> Add33/2
  t24/1 -> Add23/2
  Add23/1 -> Add9/2
  tt7/1 -> Add31/1, Add17/2
  In9/1 -> Add31/2
  In5/1 -> Add26/2, huituixinhao/4(macayali)
  Add26/1 -> Multiport Switch2/3
  con/1 -> Triggered Subsystem2/Trigger, Add33/1, Add11/1
  Triggered Subsystem2/1(force-single1) -> Add22/1
  Clock1/1 -> Add22/2
  Product1/1 -> Saturation2/1
  Add1/1 -> Product1/2
  t1/1 -> Divide2/1
  Divide2/1 -> Product1/1
  t10/1 -> Switch1/1
  t11/1 -> Switch1/3
  Add3/1 -> Switch1/2
  t12/1 -> Multiport Switch1/2
  Add4/1 -> Multiport Switch1/1
  Switch1/1 -> Add4/1
  t13/1 -> Add4/2
  Multiport Switch1/1 -> Product2/1
  Saturation2/1 -> Product2/2
  Add5/1 -> Divide2/2
  In2/1 -> Add7/1, Add5/1, Add3/2, Add1/1
  In3/1 -> Add14/2, Add26/1
  Product3/1 -> Saturation3/1
  Add2/1 -> Product3/2
  t17/1 -> Divide3/1
  Divide3/1 -> Product3/1
  t18/1 -> Switch2/1
  t19/1 -> Switch2/3
  Add6/1 -> Switch2/2
  t20/1 -> Multiport Switch2/2
  Add8/1 -> Multiport Switch2/1
  Switch2/1 -> Add8/1
  t21/1 -> Add8/2
  Multiport Switch2/1 -> Product6/1
  Saturation3/1 -> Product6/2
  Add9/1 -> Divide3/2
  In4/1 -> Add2/1, Add23/1, Add9/1, Add6/2
  Product6/1 -> Add10/3
  Product2/1 -> Add10/2
  c7/1 -> Switch5/1
  c8/1 -> Switch5/3
  Add16/1 -> Switch5/2
  Equal To Constant9/1 -> Logical Operator4/2
  Equal To Constant8/1 -> Logical Operator4/1
  tingzhendaowei/1 -> Equal To Constant9/1, Equal To Constant1/1
  Logical Operator4/1 -> huituixinhao/1(con1)
  In6/1 -> Add17/1
  Add31/1 -> huituixinhao/3(jianyashijian)
  Add17/1 -> huituixinhao/5(baoyashijian)
  In10/1 -> huituixinhao/6(zuihou;i)
  In7/1 -> huituixinhao/2(dingduanyali)
  huituixinhao/1(Out2) -> Add10/4  "weiyixinhao"
  t3/1 -> Add11/2
  t4/1 -> Multiport Switch3/2
  Switch5/1 -> Multiport Switch3/3
  suoduanliang/1 -> Add16/1
  suoduanliangsheding/1 -> Add16/2
  Multiport Switch3/1 -> Equal To Constant2/1
  Equal To Constant1/1 -> Logical Operator1/2
  Equal To Constant2/1 -> Logical Operator1/1
  Logical Operator1/1 -> Triggered Subsystem1/Trigger
  Add11/1 -> Multiport Switch3/1
  Triggered Subsystem1/1(tingzhenxinhao) -> tingzhenxinhao/1, Equal To Constant8/1

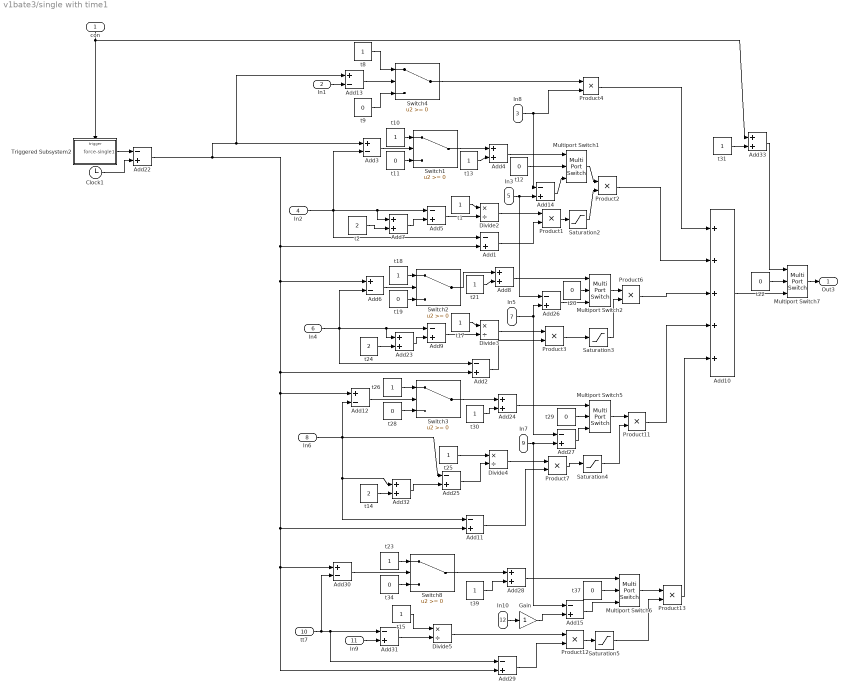
== system v1bate3/single with time1 ==
  con : Inport
  In1 : Inport  Port=2
  In8 : Inport  Port=3
  In2 : Inport  Port=4
  In3 : Inport  Port=5
  In4 : Inport  Port=6
  In5 : Inport  Port=7
  In6 : Inport  Port=8
  In7 : Inport  Port=9
  tt7 : Inport  Port=10
  In9 : Inport  Port=11
  In10 : Inport  Port=12
  Add{1..2,5,9,11,14..15,22,25..27,29,31} (13 alike) : Sum  Inputs=-+
  Add10 : Sum  Inputs=+++++
  Add{3,6,12..13,30} (5 alike) : Sum  Inputs=+-
  Add{4,7..8,23..24,28,32..33} (8 alike) : Sum
  Clock1 : Clock
  Divide{2..5} (4 alike) : Product  Inputs=*/
  Gain : Gain
  Multiport Switch{1..2,5..7} (5 alike) : MultiPortSwitch  Inputs=2
  Product{1..3,6..7,11..13} (8 alike) : Product  RndMeth=Zero
  Product4 : Product  SaturateOnIntegerOverflow=on  OutDataTypeStr=Inherit: Same as first input
  Saturation{2..5} (4 alike) : Saturate  UpperLimit=1  LowerLimit=-1
  Switch{1..4,8} (5 alike) : Switch
  Triggered Subsystem2 : Subsystem  TreatAsAtomicUnit=on
  t{1,8,10,13,15,17..18,21,23,25..26,30..31,39} (14 alike) : Constant
  t{9,11..12,19..20,22,28..29,34,37} (10 alike) : Constant  Value=0
  t14 : Constant  Value=2
  t2 : Constant  Value=2
  t24 : Constant  Value=2
  Out3 : Outport
  wires:
  In6/1 -> Add12/2, Add25/1, Add32/1, Add11/1
  Add25/1 -> Divide4/2
  Saturation4/1 -> Product11/2
  Multiport Switch5/1 -> Product11/1
  t30/1 -> Add24/2
  Switch3/1 -> Add24/1
  Add24/1 -> Multiport Switch5/1
  t29/1 -> Multiport Switch5/2
  Add12/1 -> Switch3/2
  t28/1 -> Switch3/3
  t26/1 -> Switch3/1
  Divide4/1 -> Product7/1
  t25/1 -> Divide4/1
  Add11/1 -> Product7/2
  Product7/1 -> Saturation4/1
  Product2/1 -> Add10/2
  Product6/1 -> Add10/3
  In4/1 -> Add6/2, Add9/1, Add23/1, Add2/1
  Add9/1 -> Divide3/2
  Saturation3/1 -> Product6/2
  Multiport Switch2/1 -> Product6/1
  t21/1 -> Add8/2
  Switch2/1 -> Add8/1
  Add8/1 -> Multiport Switch2/1
  t20/1 -> Multiport Switch2/2
  Add6/1 -> Switch2/2
  t19/1 -> Switch2/3
  t18/1 -> Switch2/1
  Divide3/1 -> Product3/1
  t17/1 -> Divide3/1
  Add2/1 -> Product3/2
  Product3/1 -> Saturation3/1
  In3/1 -> Add26/1, Add14/2
  In2/1 -> Add3/2, Add5/1, Add7/1, Add1/1
  Add5/1 -> Divide2/2
  Saturation2/1 -> Product2/2
  Multiport Switch1/1 -> Product2/1
  t13/1 -> Add4/2
  Switch1/1 -> Add4/1
  Add4/1 -> Multiport Switch1/1
  t12/1 -> Multiport Switch1/2
  Add3/1 -> Switch1/2
  t11/1 -> Switch1/3
  t10/1 -> Switch1/1
  Divide2/1 -> Product1/1
  t1/1 -> Divide2/1
  Add1/1 -> Product1/2
  Product1/1 -> Saturation2/1
  Clock1/1 -> Add22/2
  Triggered Subsystem2/1(force-single1) -> Add22/1
  con/1 -> Triggered Subsystem2/Trigger, Add33/1
  Add26/1 -> Multiport Switch2/3
  In5/1 -> Add27/1, Add26/2
  In7/1 -> Add27/2, Add15/1
  Add27/1 -> Multiport Switch5/3
  Add31/1 -> Divide5/2
  t39/1 -> Add28/2
  Switch8/1 -> Add28/1
  In9/1 -> Add31/2
  Add29/1 -> Product12/2
  Divide5/1 -> Product12/1
  Add28/1 -> Multiport Switch6/1
  t37/1 -> Multiport Switch6/2
  Add30/1 -> Switch8/2
  t34/1 -> Switch8/3
  t23/1 -> Switch8/1
  Multiport Switch6/1 -> Product13/1
  Saturation5/1 -> Product13/2
  Product12/1 -> Saturation5/1
  t15/1 -> Divide5/1
  tt7/1 -> Add31/1, Add29/1, Add30/2
  Product11/1 -> Add10/4
  Add23/1 -> Add9/2
  t24/1 -> Add23/2
  Add32/1 -> Add25/2
  t14/1 -> Add32/2
  t31/1 -> Add33/2
  Multiport Switch7/1 -> Out3/1
  Add33/1 -> Multiport Switch7/1
  t22/1 -> Multiport Switch7/2
  Add10/1 -> Multiport Switch7/3
  Add22/1 -> Add12/1, Add11/2, Add29/2, Add30/1, Add2/2, Add6/1, Add1/2, Add3/1, Add13/1
  Product13/1 -> Add10/5
  Add7/1 -> Add5/2
  t2/1 -> Add7/2
  t8/1 -> Switch4/1
  t9/1 -> Switch4/3
  Add13/1 -> Switch4/2
  Switch4/1 -> Product4/1
  Product4/1 -> Add10/1
  In1/1 -> Add13/2
  In8/1 -> Product4/2, Add14/1
  Add14/1 -> Multiport Switch1/3
  Add15/1 -> Multiport Switch6/3
  In10/1 -> Gain/1
  Gain/1 -> Add15/2

== system v1bate3/tvc_filter1 ==
  note: m/s2
  note: m
  In1 : Inport
  Gain : Gain  Gain=20/0.2  SaturateOnIntegerOverflow=on  OutDataTypeStr=Inherit: Same as input  ParamDataTypeStr=Inherit: Same as input
  Sum : Sum  Inputs=+++  SaturateOnIntegerOverflow=on
  Sum3 : Sum  Inputs=|++  SaturateOnIntegerOverflow=on
  acc_cal : Gain  SaturateOnIntegerOverflow=on  OutDataTypeStr=Inherit: Same as input  ParamDataTypeStr=Inherit: Same as input
  acc_ms2 : Gain  Gain=[9.8]  SaturateOnIntegerOverflow=on  OutDataTypeStr=Inherit: Same as input  ParamDataTypeStr=Inherit: Same as input
  filter : Subsystem
      mask Display: disp('x_filter')
  over_flow : RandomNumber  Variance=1e-10  SampleTime=0
  x_kar : Gain  Gain=0.0035  SaturateOnIntegerOverflow=on  OutDataTypeStr=Inherit: Same as input  ParamDataTypeStr=Inherit: Same as input
  x_kdr : Gain  SaturateOnIntegerOverflow=on  OutDataTypeStr=Inherit: Same as input  ParamDataTypeStr=Inherit: Same as input
  x_kvr : Gain  Gain=0.74  SaturateOnIntegerOverflow=on  OutDataTypeStr=Inherit: Same as input  ParamDataTypeStr=Inherit: Same as input
  x : Outport
  wires:
  over_flow/1 -> Sum3/2
  In1/1 -> acc_ms2/1
  Sum3/1 -> acc_cal/1
  acc_ms2/1 -> Sum3/1
  acc_cal/1 -> filter/1(uxa)
  x_kdr/1 -> Sum/3
  x_kvr/1 -> Sum/2
  x_kar/1 -> Sum/1
  filter/1(ax) -> x_kar/1
  filter/2(vx) -> x_kvr/1
  filter/3(dx) -> Gain/1
  Sum/1 -> x/1
  Gain/1 -> x_kdr/1

== system v1bate3/zero_position_tune1 ==
  error_in : Inport
  status : Inport  Port=2
  Gain1 : Gain  Gain=0.2  SaturateOnIntegerOverflow=on  OutDataTypeStr=Inherit: Same as input  ParamDataTypeStr=Inherit: Same as input
  Gain2 : Gain  Gain=0.001  SaturateOnIntegerOverflow=on  OutDataTypeStr=Inherit: Same as input  ParamDataTypeStr=Inherit: Same as input
  Ground : Ground
  Relational Operator : RelationalOperator  Operator===  RndMeth=Nearest  InputSameDT=on
  Saturation1 : Saturate
  Saturation2 : Saturate  UpperLimit=0.1  LowerLimit=-0.1
  Sum11 : Sum  Inputs=|++  SaturateOnIntegerOverflow=on  InputSameDT=on  OutDataTypeStr=Inherit: Same as first input
  Switch9 : Switch  Threshold=0.5  SaturateOnIntegerOverflow=on  InputSameDT=on
  Unit Delay : UnitDelay  InitialCondition=-0.03  SampleTime=0.001
  c : Constant  OutDataTypeStr=boolean
  Out : Outport
  wires:
  Saturation1/1 -> Out/1
  Gain1/1 -> Gain2/1
  status/1 -> Relational Operator/1
  error_in/1 -> Saturation2/1
  Relational Operator/1 -> Switch9/2
  c/1 -> Relational Operator/2
  Saturation2/1 -> Switch9/1
  Ground/1 -> Switch9/3
  Switch9/1 -> Gain1/1
  Sum11/1 -> Saturation1/1, Unit Delay/1
  Gain2/1 -> Sum11/1
  Unit Delay/1 -> Sum11/2
